simulink model "Dyva"  (R2020b)
settings: Solver=VariableStepAuto  StartTime=0.0  StopTime=10.0  RelTol=1e-3
PreLoadFcn:
  | m1=100;
  | k1=50;
  | b=50;
  | k12=100;
  | m2=60;
InitFcn:
  | m1 = 100;
  | k1 = 50;
  | b = 50;
  | m2=100;
  | k12=100;
model workspace (MAT data in the model file):
  k1 = 50
  k12 = 25
  m1 = 100
  m2 = 60
settings Model: Creator=com  LastModifiedBy=com

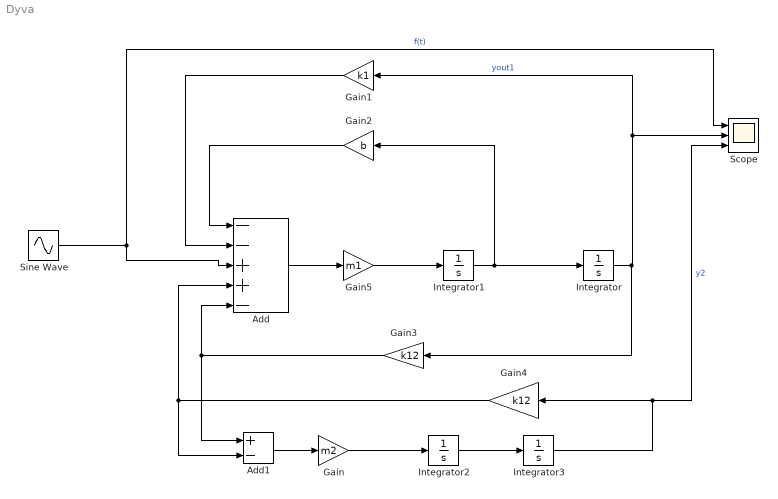
== system Dyva ==
  Add : Sum  Inputs=--++-
  Add1 : Sum  Inputs=+-
  Gain : Gain  Gain=m2
  Gain1 : Gain  Gain=k1
  Gain2 : Gain  Gain=b
  Gain3 : Gain  Gain=k12
  Gain4 : Gain  Gain=k12
  Gain5 : Gain  Gain=m1
  Integrator{,1..3} (4 alike) : Integrator
  Scope : Scope  NumInputPorts=3
  Sine Wave : Sin  Amplitude=2  Frequency=10  SampleTime=0
  wires:
  Gain2/1 -> Add/1
  Gain1/1 -> Add/2
  Add1/1 -> Gain/1
  Gain3/1 -> Add/5, Add1/1
  Gain4/1 -> Add/4, Add1/2
  Add/1 -> Gain5/1
  Gain5/1 -> Integrator1/1
  Integrator1/1 -> Gain2/1, Integrator/1
  Integrator/1 -> Gain3/1, Gain1/1, Scope/2  "yout1"
  Gain/1 -> Integrator2/1
  Integrator2/1 -> Integrator3/1
  Integrator3/1 -> Scope/3, Gain4/1  "y2"
  Sine Wave/1 -> Add/3, Scope/1  "f(t)"
